simulink model "LQR_ning"  (R2019a)
settings: Solver=FixedStepAuto  StartTime=0.0  StopTime=10  FixedStep=0.01  RelTol=1e-3
undefined symbols (not defined in the file): K, L
libraries: simulink x5, simulink_extras x1
settings Model: Creator=Ninh  LastModifiedBy=chute
settings DataIOCC: ReturnWorkspaceOutputs=off
settings DebuggingCC: ArithmeticOperatorsInVariantConditions=warning

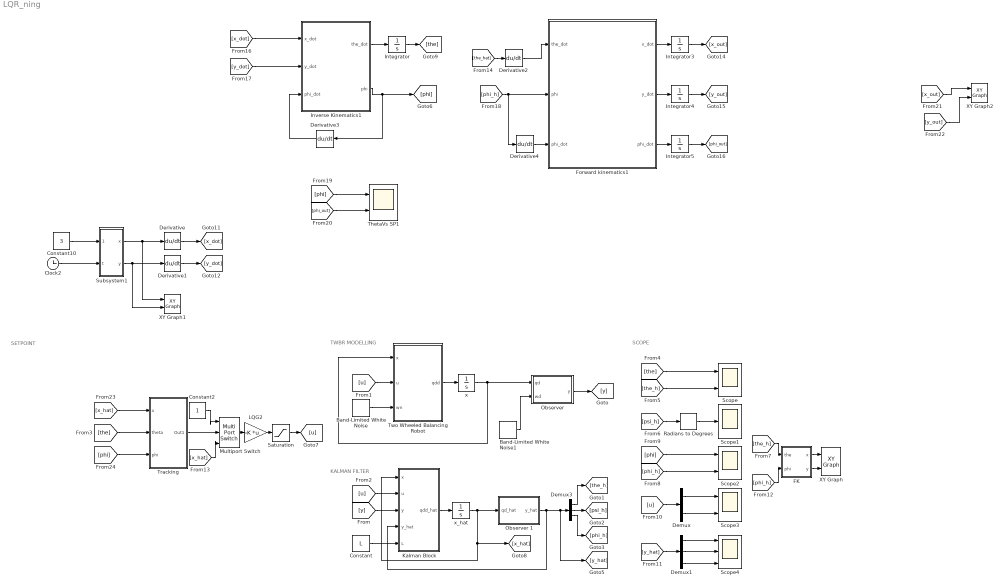
== system LQR_ning ==
  note: SCOPE
  note: SETPOINT
  note: KALMAN FILTER
  note: TWBR MODELLING
  Band-Limited White Noise : simulink/Sources/Band-Limited White Noise  Cov=[0.00000001]  Ts=0.01  seed=[1]
  Band-Limited White Noise1 : simulink/Sources/Band-Limited White Noise  Cov=[0.000000005]  Ts=0.01  seed=[1]
  Clock2 : Clock
  Constant : Constant  Value=L
  Constant10 : Constant  Value=3
  Constant2 : Constant
  Demux : Demux  Outputs=2
  Demux1 : Demux  Outputs=3
  Demux3 : Demux  Outputs=3
  Derivative{,1..4} (5 alike) : Derivative
  FK : MATLAB Function  TreatAsAtomicUnit=on
  Forward kinematics1 : MATLAB Function  TreatAsAtomicUnit=on
  Integrator : Integrator
  Integrator3 : Integrator
  Integrator4 : Integrator
  Integrator5 : Integrator  InitialCondition=[0;0]
  Inverse Kinematics1 : MATLAB Function  TreatAsAtomicUnit=on
  Kalman Block : MATLAB Function  TreatAsAtomicUnit=on
  LQG2 : Gain  Gain=-K  Multiplication=Matrix(K*u)
  Multiport Switch : MultiPortSwitch  Inputs=2
  "Observer " : MATLAB Function  TreatAsAtomicUnit=on
  Observer 1 : MATLAB Function  TreatAsAtomicUnit=on
  Radians to Degrees : simulink_extras/Transformations/Radians to Degrees
  Saturation : Saturate  UpperLimit=[12;12]  LowerLimit=[-12;-12]
  Scope : Scope  NumInputPorts=2
  Scope1 : Scope
  Scope2 : Scope  NumInputPorts=2
  Scope3 : Scope  NumInputPorts=2
  Scope4 : Scope  NumInputPorts=3
  Subsystem1 : Subsystem
  ThetaVs SP1 : Scope  NumInputPorts=2
  Tracking : Subsystem
  Two Wheeled Balancing Robot : MATLAB Function  TreatAsAtomicUnit=on
  XY Graph : simulink/Sinks/XY Graph  xmin=-0.5  xmax=0.5  ymin=-0.5  ymax=0.5  st=0.01
  XY Graph1 : simulink/Sinks/XY Graph  xmin=-1  xmax=1  ymin=-1  ymax=1  st=-1
  XY Graph2 : simulink/Sinks/XY Graph  xmin=-1  xmax=1  ymin=-1  ymax=1  st=-1
  x : Integrator  InitialCondition=[0;0;pi/30;0;0;0]
  x_hat : Integrator  InitialCondition=[0;0;pi/30;0;0;0]
  wires:
  x/1 -> Two Wheeled Balancing Robot/1(x), "Observer "/1(qd)
  Two Wheeled Balancing Robot/1(qdd) -> x/1
  Band-Limited White Noise/1 -> Two Wheeled Balancing Robot/3(wn)
  Kalman Block/1(qdd_hat) -> x_hat/1
  x_hat/1 -> Kalman Block/1(x), [x_hat], Observer 1/1(qd_hat)
  Observer 1/1(y_hat) -> Kalman Block/4(y_hat), [y_hat], Demux3/1
  [y] -> Kalman Block/3(y)
  "Observer "/1(y) -> [y]
  Band-Limited White Noise1/1 -> "Observer "/2(wd)
  Demux3/1 -> [the_h]
  Demux3/2 -> [psi_h]
  Demux3/3 -> [phi_h]
  [u] -> Two Wheeled Balancing Robot/2(u)
  [u] -> Kalman Block/2(u)
  [x_hat] -> Tracking/1(x)
  [the] -> Scope/1
  [the_h] -> Scope/2
  [psi_h] -> Radians to Degrees/1
  [phi_h] -> Scope2/2
  [phi] -> Scope2/1
  Demux/1 -> Scope3/1
  Demux/2 -> Scope3/2
  [u] -> Demux/1
  [y_hat] -> Demux1/1
  Demux1/1 -> Scope4/1
  Demux1/2 -> Scope4/2
  Demux1/3 -> Scope4/3
  Constant/1 -> Kalman Block/5(L)
  [the_h] -> FK/1(the)
  [phi_h] -> FK/2(phi)
  FK/1(x) -> XY Graph/1
  FK/2(y) -> XY Graph/2
  LQG2/1 -> Saturation/1
  Saturation/1 -> [u]
  Radians to Degrees/1 -> Scope1/1
  Constant2/1 -> Multiport Switch/1
  Multiport Switch/1 -> LQG2/1
  Tracking/1(Out1) -> Multiport Switch/2
  [x_hat] -> Multiport Switch/3
  [x_dot] -> Inverse Kinematics1/1(x_dot)
  Forward kinematics1/2(y_dot) -> Integrator4/1
  Forward kinematics1/3(phi_dot) -> Integrator5/1
  Inverse Kinematics1/2(phi) -> [phi], Derivative3/1
  Clock2/1 -> Subsystem1/2(t)
  [phi] -> ThetaVs SP1/1
  [phi_out] -> ThetaVs SP1/2
  Derivative3/1 -> Inverse Kinematics1/3(phi_dot)
  [y_out] -> XY Graph2/2
  Constant10/1 -> Subsystem1/1(mode)
  Integrator5/1 -> [phi_out]
  [x_out] -> XY Graph2/1
  Integrator3/1 -> [x_out]
  Derivative1/1 -> [y_dot]
  Subsystem1/1(x) -> Derivative/1, XY Graph1/1
  [y_dot] -> Inverse Kinematics1/2(y_dot)
  Forward kinematics1/1(x_dot) -> Integrator3/1
  Subsystem1/2(y) -> XY Graph1/2, Derivative1/1
  [phi_h] -> Derivative4/1, Forward kinematics1/2(phi)
  Derivative/1 -> [x_dot]
  Integrator4/1 -> [y_out]
  Inverse Kinematics1/1(the_dot) -> Integrator/1
  Integrator/1 -> [the]
  [the] -> Tracking/2(theta)
  [phi] -> Tracking/3(phi)
  [the_hat] -> Derivative2/1
  Derivative2/1 -> Forward kinematics1/1(the_dot)
  Derivative4/1 -> Forward kinematics1/3("phi_dot ")

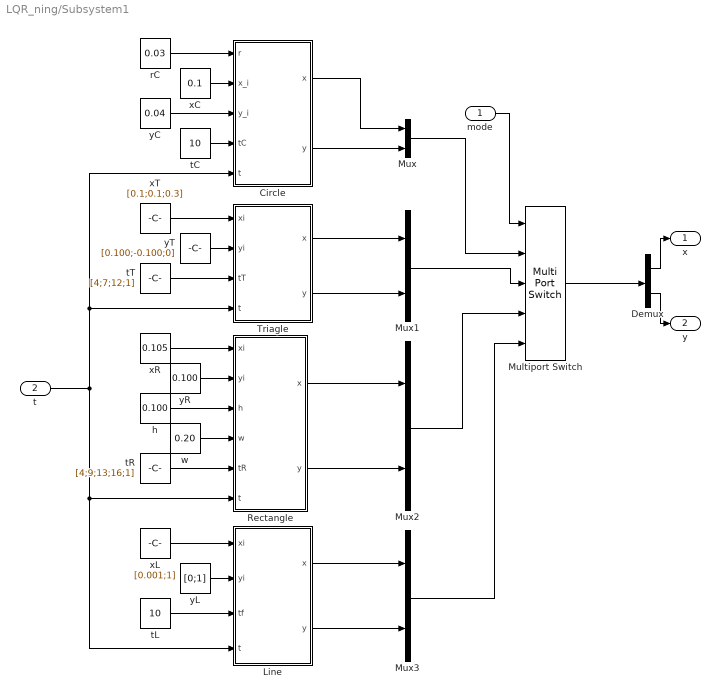
== system LQR_ning/Subsystem1 ==
  mode : Inport
  t : Inport  Port=2
  Circle : MATLAB Function  TreatAsAtomicUnit=on
  Demux : Demux  Outputs=2
  Line : MATLAB Function  TreatAsAtomicUnit=on
  Multiport Switch : MultiPortSwitch  DataPortOrder=Zero-based contiguous  Inputs=4  zeroidx=on
  Mux{,1..3} (4 alike) : Mux  Inputs=2
  Rectangle : MATLAB Function  TreatAsAtomicUnit=on
  Triagle : MATLAB Function  TreatAsAtomicUnit=on
  h : Constant  Value=0.100
  rC : Constant  Value=0.03
  tC : Constant  Value=10
  tL : Constant  Value=10
  tR : Constant  Value=[4;9;13;16;1]
  tT : Constant  Value=[4;7;12;1]
  w : Constant  Value=0.20
  xC : Constant  Value=0.1
  xL : Constant  Value=[0.001;1]
  xR : Constant  Value=0.105
  xT : Constant  Value=[0.1;0.1;0.3]
  yC : Constant  Value=0.04
  yL : Constant  Value=[0;1]
  yR : Constant  Value=0.100
  yT : Constant  Value=[0.100;-0.100;0]
  x : Outport
  y : Outport  Port=2
  wires:
  tR/1 -> Rectangle/5(tR)
  xL/1 -> Line/1(xi)
  Line/1(x) -> Mux3/1
  tC/1 -> Circle/4(tC)
  yL/1 -> Line/2(yi)
  tT/1 -> Triagle/3(tT)
  Multiport Switch/1 -> Demux/1
  Line/2(y) -> Mux3/2
  Triagle/1(x) -> Mux1/1
  Mux3/1 -> Multiport Switch/5
  xR/1 -> Rectangle/1(xi)
  Circle/2(y) -> Mux/2
  tL/1 -> Line/3(tf)
  w/1 -> Rectangle/4(w)
  Mux2/1 -> Multiport Switch/4
  mode/1 -> Multiport Switch/1
  Circle/1(x) -> Mux/1
  Mux1/1 -> Multiport Switch/3
  rC/1 -> Circle/1(r)
  Mux/1 -> Multiport Switch/2
  h/1 -> Rectangle/3(h)
  t/1 -> Circle/5(t), Triagle/4(t), Rectangle/6(t), Line/4(t)
  Demux/1 -> x/1
  xT/1 -> Triagle/1(xi)
  Rectangle/1(x) -> Mux2/1
  yT/1 -> Triagle/2(yi)
  xC/1 -> Circle/2(x_i)
  Triagle/2(y) -> Mux1/2
  yR/1 -> Rectangle/2(yi)
  Demux/2 -> y/1
  Rectangle/2(y) -> Mux2/2
  yC/1 -> Circle/3(y_i)

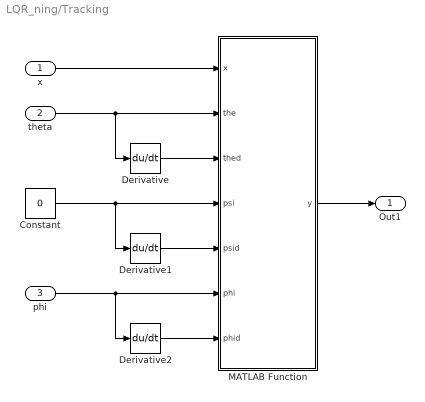
== system LQR_ning/Tracking ==
  x : Inport
  theta : Inport  Port=2
  phi : Inport  Port=3
  Constant : Constant  Value=0
  Derivative : Derivative
  Derivative1 : Derivative
  Derivative2 : Derivative
  MATLAB Function : MATLAB Function  TreatAsAtomicUnit=on
  Out1 : Outport
  wires:
  theta/1 -> Derivative/1, MATLAB Function/2(the)
  Constant/1 -> Derivative1/1, MATLAB Function/4(psi)
  phi/1 -> Derivative2/1, MATLAB Function/6(phi)
  x/1 -> MATLAB Function/1(x)
  MATLAB Function/1(y) -> Out1/1
  Derivative/1 -> MATLAB Function/3(thed)
  Derivative1/1 -> MATLAB Function/5(psid)
  Derivative2/1 -> MATLAB Function/7(phid)

== matlab function LQR_ning/Observer  ==
  data: qd input; y output; wd input
function y = fcn(qd,wd)
C = [1 0 0 0 0 0;
     0 0 1 0 0 0;
     0 0 0 0 1 0];
y = C*qd + [0;1;0]*wd;

== matlab function LQR_ning/Two Wheeled Balancing Robot ==
  data: x input; qdd output; u input; wn input
function qdd = TWBR(x,u,wn)
A =...
[        0    1.0000         0         0         0         0
         0   -0.3181   47.3795    0.3180         0         0
         0         0         0    1.0000         0         0
         0    0.1418   63.2671   -0.1418         0         0
         0         0         0         0         0    1.0000
         0         0         0         0         0   -0.4443];


B =...
[        0         0
   21.6298   21.6298
         0         0
   -9.6473   -9.6473
         0         0
  -11.6908   11.6908];
qdd = A*x + B*u + wn;

== matlab function LQR_ning/Kalman Block ==
  data: x input; u input; qdd_hat output; y input; y_hat input; L input
function qdd_hat = fcn(x,u,y,y_hat,L)
A =...
[        0    1.0000         0         0         0         0
         0   -0.3181   47.3795    0.3180         0         0
         0         0         0    1.0000         0         0
         0    0.1418   63.2671   -0.1418         0         0
         0         0         0         0         0    1.0000
         0         0         0         0         0   -0.4443];


B =...
[        0         0
   21.6298   21.6298
         0         0
   -9.6473   -9.6473
         0         0
  -11.6908   11.6908];
qdd_hat = A*x + B*u + L*(y - y_hat);

== matlab function LQR_ning/Observer 1 ==
  data: qd_hat input; y_hat output
function y_hat = fcn(qd_hat)
C = [1 0 0 0 0 0;
     0 0 1 0 0 0;
     0 0 0 0 1 0];
y_hat = C*qd_hat;

== matlab function LQR_ning/Tracking/MATLAB Function ==
  data: x input; y output; the input; thed input; psi input; psid input; phi input; phid input
function y = fcn(x,the,thed,psi,psid,phi,phid)

y = x - transpose([the,thed,psi,psid,phi,phid]);

== matlab function LQR_ning/FK ==
  data: x output; the input; y output; phi input
function [x,y]= fcn(the,phi)
R = 0.0325;
x = R*the*cos(phi);
y = R*the*sin(phi);

== matlab function LQR_ning/Forward kinematics1 ==
  data: the_dot input; x_dot output; y_dot output; phi_dot output; phi input; phi_dot input
function [x_dot,y_dot,phi_dot] = FK(the_dot,phi,phi_dot)
R =0.0335; % Wheel radius
W =0.17; % Body width
thel_dot= (the_dot-(phi_dot*W)/R);
ther_dot= the_dot+phi_dot*W/(2*R);
for i=1:1
    J=[(R/2)*cos(phi(i)),(R/2)*cos(phi(i));
       (R/2)*sin(phi(i)),(R/2)*sin(phi(i));
                     R/W,           -R/W];
end
out =J*[ther_dot;thel_dot];
x_dot=out(1,1);
y_dot =out(2,1);
phi_dot=out(3,1);
end

== matlab function LQR_ning/Inverse Kinematics1 ==
  data: x_dot input; the_dot output; y_dot input; phi_dot input; phi output
function [the_dot,phi] = fcn(x_dot,y_dot,phi_dot)

R =0.0335; % Wheel radius
W =0.17; % Body width
a=y_dot;
b=-x_dot;
d=0;
anp = atan2(b, a);
x1 = anp + atan2(sqrt(a*a + b*b - d*d), d);
phi = anp + atan2(-sqrt(a*a + b*b - d*d), d);
% =[x1;x2];
    for i=1:1
        j=(1/R)*[cos(phi(i)),sin(phi(i)),W/(2);
                 cos(phi(i)),sin(phi(i)),-W/(2)];
        out1=j*[x_dot;y_dot;phi_dot(i)];
    end
ther_dot=out1(1,1);
thel_dot=out1(2,1);

the_dot =(1/2)*(ther_dot+thel_dot);

== matlab function LQR_ning/Subsystem1/Circle ==
  data: x output; r input; x_i input; y_i input; tC input; y output; t input
% Circle
function [x,y] = fcn(r,x_i,y_i,tC,t)
t0 = 3;
if (t-t0) <=tC
    x = x_i + r*cos(2*pi*(t-t0)/tC);
    y = y_i + r*sin(2*pi*(t-t0)/tC);
else
    x = x_i + r*cos(2*pi);
    y = y_i + r*sin(2*pi);
end

== matlab function LQR_ning/Subsystem1/Line ==
  data: x output; xi input; yi input; tf input; y output; t input
% Triangle
function [x,y] = fcn(xi,yi,tf,t)
A = [xi(1);yi(1)];
B = [xi(2);yi(2)];
v0 = [0;0];
vf = [0;0];
t0=0;
if t<=tf
    Y = transpose([A v0 B vf]);
    K = [1 t0 t0^2 t0^3;
         0  1 2*t0 3*t0^2;
         1 tf tf^2 tf^3;
         0  1 2*tf 3*tf^2];
    X = inv(K)*Y;
    a = transpose(X);
    x = a(1,1) + a(1,2)*t + a(1,3)*t^2 + a(1,4)*t^3;

    y = a(2,1) + a(2,2)*t + a(2,3)*t^2 + a(2,4)*t^3;
else
    x = B(1);
    y = B(2);
end

== matlab function LQR_ning/Subsystem1/Rectangle ==
  data: x output; xi input; yi input; h input; w input; tR input; y output; t input
% rectangle
function [x,y] = fcn(xi,yi,h,w,tR,t)
x1 = xi;
x2 = xi + w;
x3 = x2;
x4 = x1;
y1 = yi;
y2 = y1;
y3 = yi - h;
y4 = y3;
A = [x1;y1];
B = [x2;y2];
C = [x3;y3];
D = [x4;y4];
v0 = [0;0];
vf = [0;0];
t0=0;t1=tR(1);t2=tR(2);t3=tR(3);tf=tR(4);
td = tR(5);
td1 = t1+td;
td2 = t2+td;
td3 = t3+td;
if t<=t1
    Y = transpose([A v0 B vf]);
    K = [1 t0 t0^2 t0^3;
         0  1 2*t0 3*t0^2;
         1 t1 t1^2 t1^3;
         0  1 2*t1 3*t1^2];
    X = inv(K)*Y;
    a = transpose(X);
    x = a(1,1) + a(1,2)*t + a(1,3)*t^2 + a(1,4)*t^3;

    y = a(2,1) + a(2,2)*t + a(2,3)*t^2 + a(2,4)*t^3;
elseif (t>t1) && (t<=td1)
    x = B(1);y = B(2);
elseif (t>td1) && (t<=t2)
    Y = transpose([B v0 C vf]);
    K = [1 td1 td1^2 td1^3;
         0  1 2*td1 3*td1^2;
         1 t2 t2^2 t2^3;
         0  1 2*t2 3*t2^2];
    X = inv(K)*Y;
    a = transpose(X);
    x = a(1,1) + a(1,2)*t + a(1,3)*t^2 + a(1,4)*t^3;

    y = a(2,1) + a(2,2)*t + a(2,3)*t^2 + a(2,4)*t^3;
elseif (t>t2) && (t<=td2)
    x = C(1);y = C(2);
elseif (t>td2) && (t<=t3)
    Y = transpose([C v0 D vf]);
    K = [1 td2 td2^2 td2^3;
         0  1 2*td2 3*td2^2;
         1 t3 t3^2 t3^3;
         0  1 2*t3 3*t3^2];
    X = inv(K)*Y;
    a = transpose(X);
    x = a(1,1) + a(1,2)*t + a(1,3)*t^2 + a(1,4)*t^3;

    y = a(2,1) + a(2,2)*t + a(2,3)*t^2 + a(2,4)*t^3;
elseif (t>t3) && (t<=td3)
    x = D(1);y = D(2);
elseif (t>td3) && (t<=tf)
    Y = transpose([D v0 A vf]);
    K = [1 td3 td3^2 td3^3;
         0  1 2*td3 3*td3^2;
         1 tf tf^2 tf^3;
         0  1 2*tf 3*tf^2];
    X = inv(K)*Y;
    a = transpose(X);
    x = a(1,1) + a(1,2)*t + a(1,3)*t^2 + a(1,4)*t^3;

    y = a(2,1) + a(2,2)*t + a(2,3)*t^2 + a(2,4)*t^3;
else
    x = A(1);
    y = A(2);
end

== matlab function LQR_ning/Subsystem1/Triagle ==
  data: x output; xi input; yi input; tT input; y output; t input
% Triangle
function [x,y] = fcn(xi,yi,tT,t)
A = [xi(1);yi(1)];
B = [xi(2);yi(2)];
C = [xi(3);yi(3)];
v0 = [0;0];
vf = [0;0];
t0=0;t1=tT(1);t2=tT(2);tf=tT(3);td = tT(1) + tT(4); tdd = tT(2) + tT(4);
if t<=t1
    Y = transpose([A v0 B vf]);
    K = [1 t0 t0^2 t0^3;
         0  1 2*t0 3*t0^2;
         1 t1 t1^2 t1^3;
         0  1 2*t1 3*t1^2];
    X = inv(K)*Y;
    a = transpose(X);
    x = a(1,1) + a(1,2)*t + a(1,3)*t^2 + a(1,4)*t^3;

    y = a(2,1) + a(2,2)*t + a(2,3)*t^2 + a(2,4)*t^3;
elseif (t>t1) && (t<=td)
    x = B(1);y = B(2);
elseif (t>td) && (t<=t2)
    Y = transpose([B v0 C vf]);
    K = [1 td td^2 td^3;
         0  1 2*td 3*td^2;
         1 t2 t2^2 t2^3;
         0  1 2*t2 3*t2^2];
    X = inv(K)*Y;
    a = transpose(X);
    x = a(1,1) + a(1,2)*t + a(1,3)*t^2 + a(1,4)*t^3;

    y = a(2,1) + a(2,2)*t + a(2,3)*t^2 + a(2,4)*t^3;
elseif (t>t2) && (t<=tdd)
    x = C(1);y = C(2);
elseif (t>tdd) && (t<=tf)
    Y = transpose([C v0 A vf]);
    K = [1 tdd tdd^2 tdd^3;
         0  1 2*tdd 3*tdd^2;
         1 tf tf^2 tf^3;
         0  1 2*tf 3*tf^2];
    X = inv(K)*Y;
    a = transpose(X);
    x = a(1,1) + a(1,2)*t + a(1,3)*t^2 + a(1,4)*t^3;

    y = a(2,1) + a(2,2)*t + a(2,3)*t^2 + a(2,4)*t^3;
else
    x = A(1);y = A(2);
end
